simulink model "sampleModel1403"  (R2023a)
settings: Solver=VariableStepAuto  StartTime=0.0  StopTime=10.0  RelTol=1e-3
libraries: simulink x5, hdlsllib x3
settings Model: Creator=user1  LastModifiedBy=user1

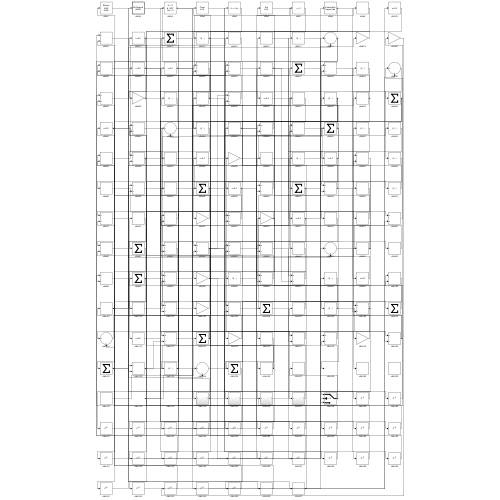
[thumbnail: Simulink's stored preview of the top-level diagram]
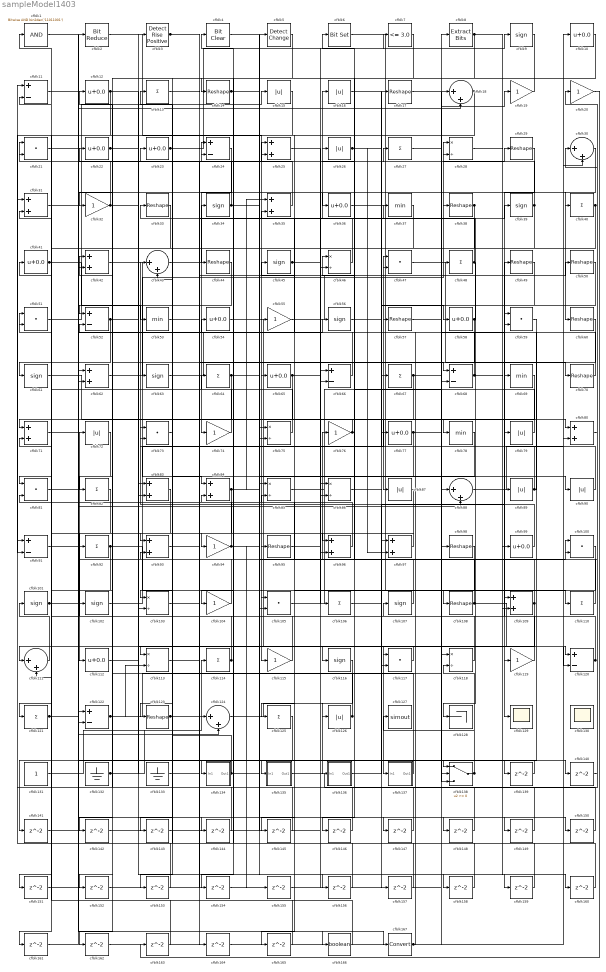
== system sampleModel1403 ==
  cfblk1 : simulink/Logic and Bit Operations/Bitwise Operator  logicop=AND  UseBitMask=on  BitMask=bin2dec('11011001')  BitMaskRealWorld=Stored Integer
      settings: LibrarySourceBlock=|
      | hdlsllib/Logic and Bit
      | Operations/Bitwise
      | Operator
  cfblk{10,12,22..23,36,41,54,58,65,77,99,112} (12 alike) : Bias  Bias=0.0  SaturateOnIntegerOverflow=off
  cfblk{21,47,51,59,73,81,100,105,117} (9 alike) : DotProduct  OutDataTypeStr=Inherit: Inherit via internal rule
  cfblk{9,34,39,45,56,61,63,101..102,107,116} (11 alike) : Signum
  cfblk{28,46,75,85..86,103,113,118} (8 alike) : Product  Inputs=*/  RndMeth=Zero  SaturateOnIntegerOverflow=on
  cfblk{19..20,32,55,74,76,94,104,115,119} (10 alike) : Gain
  cfblk{13,27,40,48,64,67,82,92,106,110,114,121,125} (13 alike) : Sum  Inputs=+
  cfblk{14,17,29,33,38,44,49..50,57,60,70,95,98,108,123} (15 alike) : Reshape
  cfblk{25,31,35,42,62,71,80,83..84,93,96..97,109} (13 alike) : Sum
  cfblk{11,24,52,66,68,91,120,122} (8 alike) : Sum  Inputs=+-
  cfblk{18,30,43,88,111,124} (6 alike) : Sum  Inputs=|++
  cfblk{15..16,26,72,79,87,89..90,126} (9 alike) : Abs  SaturateOnIntegerOverflow=off
  cfblk127 : ToWorkspace  VariableName=simout  SaveFormat=Timeseries  SampleTime=-1
  cfblk128 : Terminator
  cfblk129 : Scope
  cfblk130 : Scope
      settings: Floating=on
  cfblk131 : Constant  SampleTime=-1
  cfblk132 : Ground
  cfblk133 : Ground
  cfblk134 : Subsystem
      settings: LibrarySourceBlock=|
      | hdlsllib/Ports &
      | Subsystems/Subsystem
  cfblk135 : Subsystem
      settings: LibrarySourceBlock=|
      | hdlsllib/Ports &
      | Subsystems/Subsystem
  cfblk136 : Subsystem
      settings: LibrarySourceBlock=|
      | hdlsllib/Ports &
      | Subsystems/Subsystem
  cfblk137 : Subsystem
      settings: LibrarySourceBlock=|
      | hdlsllib/Ports &
      | Subsystems/Subsystem
  cfblk138 : Switch  SaturateOnIntegerOverflow=off  InputSameDT=off
  cfblk{139..165} (27 alike) : Delay  SampleTime=1
  cfblk166 : DataTypeConversion  OutDataTypeStr=boolean  SaturateOnIntegerOverflow=off  RndMeth=Floor
  cfblk167 : DataTypeConversion  SaturateOnIntegerOverflow=off  RndMeth=Floor
  cfblk2 : hdlsllib/Logic and Bit Operations/Bit Reduce  mode=AND
  cfblk3 : hdlsllib/Logic and Bit Operations/Detect Rise Positive  vinit=0  OutDataTypeStr=boolean
  cfblk{37,53,69,78} (4 alike) : MinMax
  cfblk4 : simulink/Logic and Bit Operations/Bit Clear  iBit=0
      settings: LibrarySourceBlock=|
      | hdlsllib/Logic and Bit
      | Operations/Bit Clear
  cfblk5 : simulink/Logic and Bit Operations/Detect Change  vinit=0  OutDataTypeStr=boolean
      settings: LibrarySourceBlock=|
      | hdlsllib/Logic and Bit
      | Operations/Detect
      | Change
  cfblk6 : simulink/Logic and Bit Operations/Bit Set  iBit=0
      settings: LibrarySourceBlock=|
      | hdlsllib/Logic and Bit
      | Operations/Bit Set
  cfblk7 : hdlsllib/Logic and Bit Operations/Compare To Constant  relop=<=  const=3.0  OutDataTypeStr=boolean
  cfblk8 : simulink/Logic and Bit Operations/Extract Bits  bitsToExtract=Upper half  numBits=8  bitIdxRange=[0 7]  outScalingMode=Preserve fixed-point scaling
      settings: LibrarySourceBlock=|
      | hdlsllib/Logic and Bit
      | Operations/Extract Bits
  wires:
  cfblk42/1 -> cfblk84/1
  cfblk99/1 -> cfblk43/1
  cfblk114/1 -> cfblk72/1, cfblk81/2
  cfblk59/1 -> cfblk135/1(In1)
  cfblk24/1 -> cfblk74/1
  cfblk46/1 -> cfblk16/1
  cfblk126/1 -> cfblk54/1, cfblk64/1
  cfblk84/1 -> cfblk35/1, cfblk47/2, cfblk143/1, cfblk159/1
  cfblk90/1 -> cfblk73/1
  cfblk52/1 -> cfblk61/1, cfblk158/1
  cfblk131/1 -> cfblk114/1
  cfblk45/1 -> cfblk66/2, cfblk7/1
  cfblk58/1 -> cfblk38/1, cfblk152/1
  cfblk123/1 -> cfblk23/1, cfblk150/1
  cfblk9/1 -> cfblk104/1
  cfblk62/1 -> cfblk28/1
  cfblk29/1 -> cfblk129/1
  cfblk105/1 -> cfblk8/1
  cfblk83/1 -> cfblk112/1
  cfblk6/1 -> cfblk78/1
  cfblk43/1 -> cfblk34/1
  cfblk38/1 -> cfblk86/2, cfblk153/1, cfblk154/1
  cfblk8/1 -> cfblk102/1, cfblk70/1
  cfblk74/1 -> cfblk21/1
  cfblk104/1 -> cfblk12/1
  cfblk51/1 -> cfblk15/1
  cfblk107/1 -> cfblk76/1
  cfblk35/1 -> cfblk22/1
  cfblk36/1 -> cfblk108/1
  cfblk120/1 -> cfblk49/1, cfblk107/1
  cfblk2/1 -> cfblk115/1
  cfblk67/1 -> cfblk87/1, cfblk109/2
  cfblk115/1 -> cfblk31/2
  cfblk22/1 -> cfblk120/2, cfblk144/1
  cfblk44/1 -> cfblk52/1
  cfblk47/1 -> cfblk69/1
  cfblk54/1 -> cfblk137/1(In1)
  cfblk102/1 -> cfblk47/1
  cfblk135/1(Out1) -> cfblk100/1
  cfblk1/1 -> cfblk167/1
  cfblk30/1 -> cfblk60/1
  cfblk86/1 -> cfblk97/1
  cfblk111/1 -> cfblk101/1
  cfblk96/1 -> cfblk51/1
  cfblk78/1 -> cfblk95/1
  cfblk63/1 -> cfblk5/1
  cfblk97/1 -> cfblk94/1
  cfblk33/1 -> cfblk111/1
  cfblk15/1 -> cfblk55/1
  cfblk109/1 -> cfblk46/1, cfblk151/1
  cfblk118/1 -> cfblk4/1
  cfblk82/1 -> cfblk121/1
  cfblk89/1 -> cfblk6/1, cfblk59/2
  cfblk77/1 -> cfblk59/1, cfblk93/1
  cfblk108/1 -> cfblk63/1, cfblk120/1
  cfblk116/1 -> cfblk136/1(In1)
  cfblk23/1 -> cfblk9/1, cfblk149/1
  cfblk3/1 -> cfblk68/1, cfblk109/1
  cfblk26/1 -> cfblk77/1, cfblk97/2
  cfblk72/1 -> cfblk122/2
  cfblk50/1 -> cfblk68/2
  cfblk60/1 -> cfblk82/1
  cfblk5/1 -> cfblk32/1
  cfblk137/1(Out1) -> cfblk92/1
  cfblk28/1 -> cfblk99/1
  cfblk117/1 -> cfblk116/1
  cfblk92/1 -> cfblk105/1, cfblk161/1
  cfblk39/1 -> cfblk28/2, cfblk83/2
  cfblk4/1 -> cfblk90/1
  cfblk34/1 -> cfblk24/1, cfblk139/1
  cfblk7/1 -> cfblk96/1
  cfblk134/1(Out1) -> cfblk100/2, cfblk93/2
  cfblk10/1 -> cfblk113/1
  cfblk93/1 -> cfblk119/1
  cfblk121/1 -> cfblk18/2, cfblk140/1
  cfblk119/1 -> cfblk51/2
  cfblk79/1 -> cfblk26/1
  cfblk55/1 -> cfblk50/1
  cfblk95/1 -> cfblk29/1
  cfblk138/1 -> cfblk127/1, cfblk118/2
  cfblk68/1 -> cfblk35/2, cfblk160/1
  cfblk40/1 -> cfblk65/1, cfblk103/2, cfblk75/2
  cfblk61/1 -> cfblk106/1
  cfblk41/1 -> cfblk53/1, cfblk25/1
  cfblk124/1 -> cfblk126/1
  cfblk27/1 -> cfblk79/1
  cfblk71/1 -> cfblk56/1
  cfblk31/1 -> cfblk36/1
  cfblk14/1 -> cfblk110/1, cfblk44/1
  cfblk122/1 -> cfblk98/1, cfblk113/2
  cfblk56/1 -> cfblk67/1
  cfblk37/1 -> cfblk134/1(In1)
  cfblk66/1 -> cfblk42/1
  cfblk87/1 -> cfblk123/1
  cfblk75/1 -> cfblk41/1
  cfblk88/1 -> cfblk30/2
  cfblk48/1 -> cfblk128/1, cfblk13/1
  cfblk101/1 -> cfblk62/1, cfblk25/2
  cfblk70/1 -> cfblk45/1
  cfblk85/1 -> cfblk17/1
  cfblk53/1 -> cfblk37/1
  cfblk17/1 -> cfblk138/3
  cfblk91/1 -> cfblk124/2
  cfblk21/1 -> cfblk2/1
  cfblk133/1 -> cfblk39/1
  cfblk19/1 -> cfblk14/1
  cfblk65/1 -> cfblk103/1, cfblk80/1
  cfblk94/1 -> cfblk52/2, cfblk155/1, cfblk156/1
  cfblk76/1 -> cfblk71/1, cfblk146/1
  cfblk103/1 -> cfblk117/1
  cfblk25/1 -> cfblk96/2
  cfblk113/1 -> cfblk48/1
  cfblk73/1 -> cfblk33/1
  cfblk16/1 -> cfblk58/1
  cfblk132/1 -> cfblk3/1, cfblk27/1
  cfblk136/1(Out1) -> cfblk89/1
  cfblk57/1 -> cfblk19/1
  cfblk64/1 -> cfblk75/1, cfblk162/1
  cfblk18/1 -> cfblk125/1, cfblk91/2
  cfblk49/1 -> cfblk117/2
  cfblk12/1 -> cfblk83/1, cfblk81/1
  cfblk11/1 -> cfblk88/2
  cfblk80/1 -> cfblk20/1
  cfblk110/1 -> cfblk85/2
  cfblk32/1 -> cfblk11/2, cfblk40/1
  cfblk139/1 -> cfblk138/1
  cfblk140/1 -> cfblk30/1
  cfblk125/1 -> cfblk141/1
  cfblk69/1 -> cfblk142/1
  cfblk142/1 -> cfblk105/2
  cfblk143/1 -> cfblk66/1
  cfblk144/1 -> cfblk73/2
  cfblk100/1 -> cfblk145/1
  cfblk145/1 -> cfblk21/2
  cfblk146/1 -> cfblk85/1
  cfblk112/1 -> cfblk147/1
  cfblk147/1 -> cfblk84/2
  cfblk81/1 -> cfblk148/1
  cfblk148/1 -> cfblk11/1
  cfblk149/1 -> cfblk71/2
  cfblk150/1 -> cfblk42/2
  cfblk151/1 -> cfblk124/1
  cfblk152/1 -> cfblk88/1
  cfblk153/1 -> cfblk31/1
  cfblk154/1 -> cfblk46/2
  cfblk155/1 -> cfblk18/1
  cfblk156/1 -> cfblk91/1
  cfblk106/1 -> cfblk157/1
  cfblk157/1 -> cfblk43/2
  cfblk158/1 -> cfblk86/1
  cfblk159/1 -> cfblk24/2
  cfblk160/1 -> cfblk138/2
  cfblk161/1 -> cfblk62/2
  cfblk162/1 -> cfblk118/1
  cfblk20/1 -> cfblk163/1
  cfblk163/1 -> cfblk111/2
  cfblk13/1 -> cfblk164/1
  cfblk164/1 -> cfblk10/1
  cfblk98/1 -> cfblk165/1
  cfblk165/1 -> cfblk122/1
  cfblk141/1 -> cfblk166/1
  cfblk166/1 -> cfblk1/1
  cfblk167/1 -> cfblk80/2, cfblk57/1

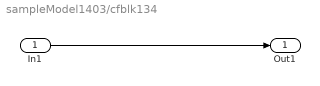
== system sampleModel1403/cfblk134 ==
  In1 : Inport
  Out1 : Outport
  wires:
  In1/1 -> Out1/1

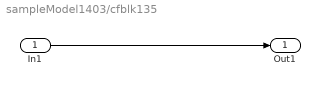
== system sampleModel1403/cfblk135 ==
  In1 : Inport
  Out1 : Outport
  wires:
  In1/1 -> Out1/1

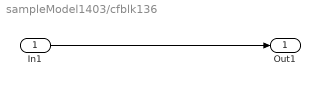
== system sampleModel1403/cfblk136 ==
  In1 : Inport
  Out1 : Outport
  wires:
  In1/1 -> Out1/1

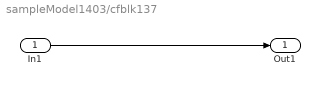
== system sampleModel1403/cfblk137 ==
  In1 : Inport
  Out1 : Outport
  wires:
  In1/1 -> Out1/1
